simulink model "TopLevelModel"  (R2023a)
settings: Solver=VariableStepAuto  StartTime=0.0  StopTime=inf  RelTol=1e-3
values from neighbouring files (symbols this model uses):
  b = 40.6518    [TopLevelModelParameters.m]
  B1 = 0.0042    [TopLevelModelParameters.m]
  B2 = 0.0084    [TopLevelModelParameters.m]
  J1 = 7e-5    (= 7e-05)    [TopLevelModelParameters.m]
  J2 = 8e-5    (= 8e-05)    [TopLevelModelParameters.m]
  k1 = 2.6552e5    (= 265520)    [TopLevelModelParameters.m]
  k2 = 2.6552e5    (= 265520)    [TopLevelModelParameters.m]
  k3 = 11.777e4    (= 117770)    [TopLevelModelParameters.m]
  Kb = 23e-3    (= 0.023)    [TopLevelModelParameters.m]
  Kt = 23e-3    (= 0.023)    [TopLevelModelParameters.m]
  L = 0.1    [TopLevelModelParameters.m]
  m = 2    [TopLevelModelParameters.m]
  R = 0.71    [TopLevelModelParameters.m]
  r = 0.0194    [TopLevelModelParameters.m]
undefined symbols (not defined in the file or in its folder): J, Kd, Ke
libraries: fl_lib x40, fl_ps_legacy_lib x16, nesl_utility x12, slpidlib x10, SignalEditorBlockLib x4, ee_lib x4, simulink x2
(part 3 of 3)

== system TopLevelModel/Belt2/Subsystem2/Subsystem ==
  Constant : Constant  Value=Kt
  Constant1 : Constant  Value=Ke
  Constant2 : Constant  Value=R
  Divide : Product  Inputs=**/
  Divide1 : Product  Inputs=***/
  Minus3 : Sum  Inputs=+-
  Voltage : DiscretePulseGenerator  PulseType=Time based  Amplitude=12  Period=11  PulseWidth=50  PhaseDelay=2
  Tourque : Outport
  wires:
  Divide1/1 -> Minus3/2
  Divide/1 -> Minus3/1
  Constant/1 -> Divide/2, Divide1/1
  [theta1_dot] -> Divide1/3
  Constant1/1 -> Divide1/2
  Constant2/1 -> Divide1/4, Divide/3
  Minus3/1 -> Tourque/1  "Tourque"
  Voltage/1 -> Divide/1

== system TopLevelModel/Belt3/Subsystem2/DC Motor1 ==
  note: Armature Controlled DC Motor
      |
      | $E_a = R_a \cdot I_a + L_a \cdot \frac{di_a}{dt} + K_b \cdot \frac{d\theta}{dt}$
      | $T_{m} = K_{t} \cdot I_{a}$
  Voltage : Inport
  Velocity : Inport  Port=2
  Constant1 : Constant  Value=R
  Gain1 : Gain  Gain=Kb
  Gain2 : Gain  Gain=1/L
  Gain3 : Gain  Gain=Kt
  Integrator : Integrator
  Product : Product
  Subtract : Sum  Inputs=+--
  Tourque : Outport
  wires:
  Voltage/1 -> Subtract/1
  Integrator/1 -> Product/1, Gain3/1  "i"
  Gain3/1 -> Tourque/1
  Gain1/1 -> Subtract/2
  Velocity/1 -> Gain1/1
  Constant1/1 -> Product/2
  Product/1 -> Subtract/3
  Gain2/1 -> Integrator/1  "i_dot"
  Subtract/1 -> Gain2/1

== system TopLevelModel/Belt3/Subsystem2/Subsystem ==
  Constant : Constant  Value=Kt
  Constant1 : Constant  Value=Ke
  Constant2 : Constant  Value=R
  Divide : Product  Inputs=**/
  Divide1 : Product  Inputs=***/
  Minus3 : Sum  Inputs=+-
  Voltage : DiscretePulseGenerator  PulseType=Time based  Amplitude=12  Period=11  PulseWidth=50  PhaseDelay=2
  Tourque : Outport
  wires:
  Divide1/1 -> Minus3/2
  Divide/1 -> Minus3/1
  Constant/1 -> Divide/2, Divide1/1
  [theta1_dot] -> Divide1/3
  Constant1/1 -> Divide1/2
  Constant2/1 -> Divide1/4, Divide/3
  Minus3/1 -> Tourque/1  "Tourque"
  Voltage/1 -> Divide/1

== system TopLevelModel/Belt4/Subsystem2/DC Motor1 ==
  note: Armature Controlled DC Motor
      |
      | $E_a = R_a \cdot I_a + L_a \cdot \frac{di_a}{dt} + K_b \cdot \frac{d\theta}{dt}$
      | $T_{m} = K_{t} \cdot I_{a}$
  Voltage : Inport
  Velocity : Inport  Port=2
  Constant1 : Constant  Value=R
  Gain1 : Gain  Gain=Kb
  Gain2 : Gain  Gain=1/L
  Gain3 : Gain  Gain=Kt
  Integrator : Integrator
  Product : Product
  Subtract : Sum  Inputs=+--
  Tourque : Outport
  wires:
  Voltage/1 -> Subtract/1
  Integrator/1 -> Product/1, Gain3/1  "i"
  Gain3/1 -> Tourque/1
  Gain1/1 -> Subtract/2
  Velocity/1 -> Gain1/1
  Constant1/1 -> Product/2
  Product/1 -> Subtract/3
  Gain2/1 -> Integrator/1  "i_dot"
  Subtract/1 -> Gain2/1

== system TopLevelModel/Belt4/Subsystem2/Subsystem ==
  Constant : Constant  Value=Kt
  Constant1 : Constant  Value=Ke
  Constant2 : Constant  Value=R
  Divide : Product  Inputs=**/
  Divide1 : Product  Inputs=***/
  Minus3 : Sum  Inputs=+-
  Voltage : DiscretePulseGenerator  PulseType=Time based  Amplitude=12  Period=11  PulseWidth=50  PhaseDelay=2
  Tourque : Outport
  wires:
  Divide1/1 -> Minus3/2
  Divide/1 -> Minus3/1
  Constant/1 -> Divide/2, Divide1/1
  [theta1_dot] -> Divide1/3
  Constant1/1 -> Divide1/2
  Constant2/1 -> Divide1/4, Divide/3
  Minus3/1 -> Tourque/1  "Tourque"
  Voltage/1 -> Divide/1

== system TopLevelModel/Belt5/Subsystem2/DC Motor1 ==
  note: Armature Controlled DC Motor
      |
      | $E_a = R_a \cdot I_a + L_a \cdot \frac{di_a}{dt} + K_b \cdot \frac{d\theta}{dt}$
      | $T_{m} = K_{t} \cdot I_{a}$
  Voltage : Inport
  Velocity : Inport  Port=2
  Constant1 : Constant  Value=R
  Gain1 : Gain  Gain=Kb
  Gain2 : Gain  Gain=1/L
  Gain3 : Gain  Gain=Kt
  Integrator : Integrator
  Product : Product
  Subtract : Sum  Inputs=+--
  Tourque : Outport
  wires:
  Voltage/1 -> Subtract/1
  Integrator/1 -> Product/1, Gain3/1  "i"
  Gain3/1 -> Tourque/1
  Gain1/1 -> Subtract/2
  Velocity/1 -> Gain1/1
  Constant1/1 -> Product/2
  Product/1 -> Subtract/3
  Gain2/1 -> Integrator/1  "i_dot"
  Subtract/1 -> Gain2/1

== system TopLevelModel/Belt5/Subsystem2/Subsystem ==
  Constant : Constant  Value=Kt
  Constant1 : Constant  Value=Ke
  Constant2 : Constant  Value=R
  Divide : Product  Inputs=**/
  Divide1 : Product  Inputs=***/
  Minus3 : Sum  Inputs=+-
  Voltage : DiscretePulseGenerator  PulseType=Time based  Amplitude=12  Period=11  PulseWidth=50  PhaseDelay=2
  Tourque : Outport
  wires:
  Divide1/1 -> Minus3/2
  Divide/1 -> Minus3/1
  Constant/1 -> Divide/2, Divide1/1
  [theta1_dot] -> Divide1/3
  Constant1/1 -> Divide1/2
  Constant2/1 -> Divide1/4, Divide/3
  Minus3/1 -> Tourque/1  "Tourque"
  Voltage/1 -> Divide/1

== system TopLevelModel/Belt6/Subsystem2/DC Motor1 ==
  note: Armature Controlled DC Motor
      |
      | $E_a = R_a \cdot I_a + L_a \cdot \frac{di_a}{dt} + K_b \cdot \frac{d\theta}{dt}$
      | $T_{m} = K_{t} \cdot I_{a}$
  Voltage : Inport
  Velocity : Inport  Port=2
  Constant1 : Constant  Value=R
  Gain1 : Gain  Gain=Kb
  Gain2 : Gain  Gain=1/L
  Gain3 : Gain  Gain=Kt
  Integrator : Integrator
  Product : Product
  Subtract : Sum  Inputs=+--
  Tourque : Outport
  wires:
  Voltage/1 -> Subtract/1
  Integrator/1 -> Product/1, Gain3/1  "i"
  Gain3/1 -> Tourque/1
  Gain1/1 -> Subtract/2
  Velocity/1 -> Gain1/1
  Constant1/1 -> Product/2
  Product/1 -> Subtract/3
  Gain2/1 -> Integrator/1  "i_dot"
  Subtract/1 -> Gain2/1

== system TopLevelModel/Belt6/Subsystem2/Subsystem ==
  Constant : Constant  Value=Kt
  Constant1 : Constant  Value=Ke
  Constant2 : Constant  Value=R
  Divide : Product  Inputs=**/
  Divide1 : Product  Inputs=***/
  Minus3 : Sum  Inputs=+-
  Voltage : DiscretePulseGenerator  PulseType=Time based  Amplitude=12  Period=11  PulseWidth=50  PhaseDelay=2
  Tourque : Outport
  wires:
  Divide1/1 -> Minus3/2
  Divide/1 -> Minus3/1
  Constant/1 -> Divide/2, Divide1/1
  [theta1_dot] -> Divide1/3
  Constant1/1 -> Divide1/2
  Constant2/1 -> Divide1/4, Divide/3
  Minus3/1 -> Tourque/1  "Tourque"
  Voltage/1 -> Divide/1

== system TopLevelModel/Belt7/Subsystem2/DC Motor1 ==
  note: Armature Controlled DC Motor
      |
      | $E_a = R_a \cdot I_a + L_a \cdot \frac{di_a}{dt} + K_b \cdot \frac{d\theta}{dt}$
      | $T_{m} = K_{t} \cdot I_{a}$
  Voltage : Inport
  Velocity : Inport  Port=2
  Constant1 : Constant  Value=R
  Gain1 : Gain  Gain=Kb
  Gain2 : Gain  Gain=1/L
  Gain3 : Gain  Gain=Kt
  Integrator : Integrator
  Product : Product
  Subtract : Sum  Inputs=+--
  Tourque : Outport
  wires:
  Voltage/1 -> Subtract/1
  Integrator/1 -> Product/1, Gain3/1  "i"
  Gain3/1 -> Tourque/1
  Gain1/1 -> Subtract/2
  Velocity/1 -> Gain1/1
  Constant1/1 -> Product/2
  Product/1 -> Subtract/3
  Gain2/1 -> Integrator/1  "i_dot"
  Subtract/1 -> Gain2/1

== system TopLevelModel/Belt7/Subsystem2/Subsystem ==
  Constant : Constant  Value=Kt
  Constant1 : Constant  Value=Ke
  Constant2 : Constant  Value=R
  Divide : Product  Inputs=**/
  Divide1 : Product  Inputs=***/
  Minus3 : Sum  Inputs=+-
  Voltage : DiscretePulseGenerator  PulseType=Time based  Amplitude=12  Period=11  PulseWidth=50  PhaseDelay=2
  Tourque : Outport
  wires:
  Divide1/1 -> Minus3/2
  Divide/1 -> Minus3/1
  Constant/1 -> Divide/2, Divide1/1
  [theta1_dot] -> Divide1/3
  Constant1/1 -> Divide1/2
  Constant2/1 -> Divide1/4, Divide/3
  Minus3/1 -> Tourque/1  "Tourque"
  Voltage/1 -> Divide/1

== system TopLevelModel/Belt8/Subsystem2/DC Motor1 ==
  note: Armature Controlled DC Motor
      |
      | $E_a = R_a \cdot I_a + L_a \cdot \frac{di_a}{dt} + K_b \cdot \frac{d\theta}{dt}$
      | $T_{m} = K_{t} \cdot I_{a}$
  Voltage : Inport
  Velocity : Inport  Port=2
  Constant1 : Constant  Value=R
  Gain1 : Gain  Gain=Kb
  Gain2 : Gain  Gain=1/L
  Gain3 : Gain  Gain=Kt
  Integrator : Integrator
  Product : Product
  Subtract : Sum  Inputs=+--
  Tourque : Outport
  wires:
  Voltage/1 -> Subtract/1
  Integrator/1 -> Product/1, Gain3/1  "i"
  Gain3/1 -> Tourque/1
  Gain1/1 -> Subtract/2
  Velocity/1 -> Gain1/1
  Constant1/1 -> Product/2
  Product/1 -> Subtract/3
  Gain2/1 -> Integrator/1  "i_dot"
  Subtract/1 -> Gain2/1

== system TopLevelModel/Belt8/Subsystem2/Subsystem ==
  Constant : Constant  Value=Kt
  Constant1 : Constant  Value=Ke
  Constant2 : Constant  Value=R
  Divide : Product  Inputs=**/
  Divide1 : Product  Inputs=***/
  Minus3 : Sum  Inputs=+-
  Voltage : DiscretePulseGenerator  PulseType=Time based  Amplitude=12  Period=11  PulseWidth=50  PhaseDelay=2
  Tourque : Outport
  wires:
  Divide1/1 -> Minus3/2
  Divide/1 -> Minus3/1
  Constant/1 -> Divide/2, Divide1/1
  [theta1_dot] -> Divide1/3
  Constant1/1 -> Divide1/2
  Constant2/1 -> Divide1/4, Divide/3
  Minus3/1 -> Tourque/1  "Tourque"
  Voltage/1 -> Divide/1

== system TopLevelModel/Belt9/Subsystem2/DC Motor1 ==
  note: Armature Controlled DC Motor
      |
      | $E_a = R_a \cdot I_a + L_a \cdot \frac{di_a}{dt} + K_b \cdot \frac{d\theta}{dt}$
      | $T_{m} = K_{t} \cdot I_{a}$
  Voltage : Inport
  Velocity : Inport  Port=2
  Constant1 : Constant  Value=R
  Gain1 : Gain  Gain=Kb
  Gain2 : Gain  Gain=1/L
  Gain3 : Gain  Gain=Kt
  Integrator : Integrator
  Product : Product
  Subtract : Sum  Inputs=+--
  Tourque : Outport
  wires:
  Voltage/1 -> Subtract/1
  Integrator/1 -> Product/1, Gain3/1  "i"
  Gain3/1 -> Tourque/1
  Gain1/1 -> Subtract/2
  Velocity/1 -> Gain1/1
  Constant1/1 -> Product/2
  Product/1 -> Subtract/3
  Gain2/1 -> Integrator/1  "i_dot"
  Subtract/1 -> Gain2/1

== system TopLevelModel/Belt9/Subsystem2/Subsystem ==
  Constant : Constant  Value=Kt
  Constant1 : Constant  Value=Ke
  Constant2 : Constant  Value=R
  Divide : Product  Inputs=**/
  Divide1 : Product  Inputs=***/
  Minus3 : Sum  Inputs=+-
  Voltage : DiscretePulseGenerator  PulseType=Time based  Amplitude=12  Period=11  PulseWidth=50  PhaseDelay=2
  Tourque : Outport
  wires:
  Divide1/1 -> Minus3/2
  Divide/1 -> Minus3/1
  Constant/1 -> Divide/2, Divide1/1
  [theta1_dot] -> Divide1/3
  Constant1/1 -> Divide1/2
  Constant2/1 -> Divide1/4, Divide/3
  Minus3/1 -> Tourque/1  "Tourque"
  Voltage/1 -> Divide/1

== system TopLevelModel/Controller/Position/Algorithm and Pulse Generation ==
  note: The reference input defines the required angular position in terms of
      | the number steps. For this stepper, the step size is 1.8 degrees. Hence
      | a demand of 10 steps results in an angle change of 18 degrees.
      | The step rate is set by the Pulse Generator's Pulse rate mask parameter.
  note: Position Controller
  Reference : Inport
  IC Analog Output REV : Subsystem
  IC Analog Output Vref : Subsystem
  Logic2Volts1 : Gain  Gain=5
  Logic2Volts2 : Gain  Gain=5
  Pulse Generator : Subsystem  mask{f=20}
      mask prompts: f "Pulse rate"
  Rate Transition : RateTransition  Deterministic=off
  REV : PMIOPort  Side=Right
  Vref : PMIOPort  Port=2  Side=Right
  wires:
  Logic2Volts1/1 -> IC Analog Output Vref/1(SL)
  Pulse Generator/1(Pulse train) -> Logic2Volts1/1
  Reference/1 -> Rate Transition/1
  Logic2Volts2/1 -> IC Analog Output REV/1(SL)
  Pulse Generator/2(Pulse direction) -> Logic2Volts2/1
  Rate Transition/1 -> Pulse Generator/1(Pulse  demand)
  connections:
  Vref/RConn1 -- IC Analog Output Vref/RConn1
  REV/RConn1 -- IC Analog Output REV/RConn1

== system TopLevelModel/Controller/Speed/Step Rate and Direction ==
  note: The speed controller turns the reference input into an absolute voltage demand for the
      | voltage-controlled pulse generator and sets the reverse flag signal to +5 volts when the
      | speed demand is negative.
  Reference : Inport
  Abs : Abs  SaturateOnIntegerOverflow=off
  Compare To Constant : simulink/Logic and Bit Operations/Compare To Constant  relop=<  const=0  OutDataTypeStr=uint8  ZeroCross=off
  Data Type Conversion : DataTypeConversion  SaturateOnIntegerOverflow=off  RndMeth=Floor
  IC Analog Output REV : Subsystem
  IC Analog Output Vref : Subsystem
  Logic2Volts : Gain  Gain=5
  Max step rate 100/s : Saturate  UpperLimit=100  LowerLimit=0
  StepRate2Volts : Gain  Gain=5/100
  REV : PMIOPort  Side=Right
  Vref : PMIOPort  Port=2  Side=Right
  wires:
  StepRate2Volts/1 -> IC Analog Output Vref/1(SL)
  Max step rate 100/s/1 -> StepRate2Volts/1
  Data Type Conversion/1 -> Logic2Volts/1
  Compare To Constant/1 -> Data Type Conversion/1
  Reference/1 -> Compare To Constant/1, Abs/1
  Abs/1 -> Max step rate 100/s/1
  Logic2Volts/1 -> IC Analog Output REV/1(SL)
  connections:
  REV/RConn1 -- IC Analog Output REV/RConn1
  Vref/RConn1 -- IC Analog Output Vref/RConn1

== system TopLevelModel/Controller/Speed/Voltage-Controlled Pulse Generator ==
  2*pi : fl_ps_legacy_lib/Legacy Physical Signals/Functions/PS Gain  gain=-2*pi
  Controlled Voltage Source : fl_lib/Electrical/Electrical Sources/Controlled Voltage Source
  ERef : fl_lib/Electrical/Electrical Elements/Electrical Reference
  Max step rate =100 : fl_ps_legacy_lib/Legacy Physical Signals/Functions/PS Gain  gain=100
  Normalize to 1 : fl_ps_legacy_lib/Legacy Physical Signals/Functions/PS Gain  gain=1/5
  PS Integrator : fl_ps_legacy_lib/Legacy Physical Signals/Linear Operators/PS Integrator  x0=0
      settings: InternalSimscapePortConfiguration="{\"Bottom\":[],\"Left\":[{\"id\":\"I\",\"label\":\"\",\"type\":\"input\"}],\"Right\":[{\"id\":\"O\",\"label\":\"\",\"type\":\"output\"}],\"Top\":[]}"
  PS Sign : fl_ps_legacy_lib/Legacy Physical Signals/Nonlinear Operators/PS Sign
      settings: InternalSimscapePortConfiguration="{\"Bottom\":[],\"Left\":[{\"id\":\"I\",\"label\":\"\",\"type\":\"input\"}],\"Right\":[{\"id\":\"O\",\"label\":\"\",\"type\":\"output\"}],\"Top\":[]}"
  PS Sine : fl_ps_legacy_lib/Legacy Physical Signals/Functions/PS Math Function  fcn_choice=1
      settings: InternalSimscapePortConfiguration="{\"Bottom\":[],\"Left\":[{\"id\":\"I\",\"label\":\"\",\"type\":\"input\"}],\"Right\":[{\"id\":\"O\",\"label\":\"\",\"type\":\"output\"}],\"Top\":[]}"
  Voltage Sensor : fl_lib/Electrical/Electrical Sensors/Voltage Sensor
  "[0,1]" : fl_ps_legacy_lib/Legacy Physical Signals/Nonlinear Operators/PS Saturation  upper_limit=1  lower_limit=0
      settings: InternalSimscapePortConfiguration="{\"Bottom\":[],\"Left\":[{\"id\":\"I\",\"label\":\"\",\"type\":\"input\"}],\"Right\":[{\"id\":\"O\",\"label\":\"\",\"type\":\"output\"}],\"Top\":[]}"
  logic2volts : fl_ps_legacy_lib/Legacy Physical Signals/Functions/PS Gain  gain=5
  PWM : PMIOPort  Side=Right
  0v : PMIOPort  Port=2  Side=Right
  Vref : PMIOPort  Port=3  Side=Left
  connections:
  PWM/RConn1 -- Controlled Voltage Source/LConn1
  Controlled Voltage Source/RConn2 -- 0v/RConn1
  Vref/RConn1 -- Voltage Sensor/LConn1
  ERef/LConn1 -- Voltage Sensor/RConn2
  Voltage Sensor/RConn1 -- Normalize to 1/LConn1
  Max step rate =100/LConn1 -- Normalize to 1/RConn1
  Max step rate =100/RConn1 -- 2*pi/LConn1
  2*pi/RConn1 -- PS Integrator/LConn1
  PS Integrator/RConn1 -- PS Sine/LConn1
  PS Sign/LConn1 -- PS Sine/RConn1
  "[0,1]"/LConn1 -- PS Sign/RConn1
  "[0,1]"/RConn1 -- logic2volts/LConn1
  logic2volts/RConn1 -- Controlled Voltage Source/RConn1

== system TopLevelModel/Controller1/Position/Algorithm and Pulse Generation ==
  note: The reference input defines the required angular position in terms of
      | the number steps. For this stepper, the step size is 1.8 degrees. Hence
      | a demand of 10 steps results in an angle change of 18 degrees.
      | The step rate is set by the Pulse Generator's Pulse rate mask parameter.
  note: Position Controller
  Reference : Inport
  IC Analog Output REV : Subsystem
  IC Analog Output Vref : Subsystem
  Logic2Volts1 : Gain  Gain=5
  Logic2Volts2 : Gain  Gain=5
  Pulse Generator : Subsystem  mask{f=20}
      mask prompts: f "Pulse rate"
  Rate Transition : RateTransition  Deterministic=off
  REV : PMIOPort  Side=Right
  Vref : PMIOPort  Port=2  Side=Right
  wires:
  Logic2Volts1/1 -> IC Analog Output Vref/1(SL)
  Pulse Generator/1(Pulse train) -> Logic2Volts1/1
  Reference/1 -> Rate Transition/1
  Logic2Volts2/1 -> IC Analog Output REV/1(SL)
  Pulse Generator/2(Pulse direction) -> Logic2Volts2/1
  Rate Transition/1 -> Pulse Generator/1(Pulse  demand)
  connections:
  Vref/RConn1 -- IC Analog Output Vref/RConn1
  REV/RConn1 -- IC Analog Output REV/RConn1

== system TopLevelModel/Controller1/Speed/Step Rate and Direction ==
  note: The speed controller turns the reference input into an absolute voltage demand for the
      | voltage-controlled pulse generator and sets the reverse flag signal to +5 volts when the
      | speed demand is negative.
  Reference : Inport
  Abs : Abs  SaturateOnIntegerOverflow=off
  Compare To Constant : simulink/Logic and Bit Operations/Compare To Constant  relop=<  const=0  OutDataTypeStr=uint8  ZeroCross=off
  Data Type Conversion : DataTypeConversion  SaturateOnIntegerOverflow=off  RndMeth=Floor
  IC Analog Output REV : Subsystem
  IC Analog Output Vref : Subsystem
  Logic2Volts : Gain  Gain=5
  Max step rate 100/s : Saturate  UpperLimit=100  LowerLimit=0
  StepRate2Volts : Gain  Gain=5/100
  REV : PMIOPort  Side=Right
  Vref : PMIOPort  Port=2  Side=Right
  wires:
  StepRate2Volts/1 -> IC Analog Output Vref/1(SL)
  Max step rate 100/s/1 -> StepRate2Volts/1
  Data Type Conversion/1 -> Logic2Volts/1
  Compare To Constant/1 -> Data Type Conversion/1
  Reference/1 -> Compare To Constant/1, Abs/1
  Abs/1 -> Max step rate 100/s/1
  Logic2Volts/1 -> IC Analog Output REV/1(SL)
  connections:
  REV/RConn1 -- IC Analog Output REV/RConn1
  Vref/RConn1 -- IC Analog Output Vref/RConn1

== system TopLevelModel/Controller1/Speed/Voltage-Controlled Pulse Generator ==
  2*pi : fl_ps_legacy_lib/Legacy Physical Signals/Functions/PS Gain  gain=-2*pi
  Controlled Voltage Source : fl_lib/Electrical/Electrical Sources/Controlled Voltage Source
  ERef : fl_lib/Electrical/Electrical Elements/Electrical Reference
  Max step rate =100 : fl_ps_legacy_lib/Legacy Physical Signals/Functions/PS Gain  gain=100
  Normalize to 1 : fl_ps_legacy_lib/Legacy Physical Signals/Functions/PS Gain  gain=1/5
  PS Integrator : fl_ps_legacy_lib/Legacy Physical Signals/Linear Operators/PS Integrator  x0=0
      settings: InternalSimscapePortConfiguration="{\"Bottom\":[],\"Left\":[{\"id\":\"I\",\"label\":\"\",\"type\":\"input\"}],\"Right\":[{\"id\":\"O\",\"label\":\"\",\"type\":\"output\"}],\"Top\":[]}"
  PS Sign : fl_ps_legacy_lib/Legacy Physical Signals/Nonlinear Operators/PS Sign
      settings: InternalSimscapePortConfiguration="{\"Bottom\":[],\"Left\":[{\"id\":\"I\",\"label\":\"\",\"type\":\"input\"}],\"Right\":[{\"id\":\"O\",\"label\":\"\",\"type\":\"output\"}],\"Top\":[]}"
  PS Sine : fl_ps_legacy_lib/Legacy Physical Signals/Functions/PS Math Function  fcn_choice=1
      settings: InternalSimscapePortConfiguration="{\"Bottom\":[],\"Left\":[{\"id\":\"I\",\"label\":\"\",\"type\":\"input\"}],\"Right\":[{\"id\":\"O\",\"label\":\"\",\"type\":\"output\"}],\"Top\":[]}"
  Voltage Sensor : fl_lib/Electrical/Electrical Sensors/Voltage Sensor
  "[0,1]" : fl_ps_legacy_lib/Legacy Physical Signals/Nonlinear Operators/PS Saturation  upper_limit=1  lower_limit=0
      settings: InternalSimscapePortConfiguration="{\"Bottom\":[],\"Left\":[{\"id\":\"I\",\"label\":\"\",\"type\":\"input\"}],\"Right\":[{\"id\":\"O\",\"label\":\"\",\"type\":\"output\"}],\"Top\":[]}"
  logic2volts : fl_ps_legacy_lib/Legacy Physical Signals/Functions/PS Gain  gain=5
  PWM : PMIOPort  Side=Right
  0v : PMIOPort  Port=2  Side=Right
  Vref : PMIOPort  Port=3  Side=Left
  connections:
  PWM/RConn1 -- Controlled Voltage Source/LConn1
  Controlled Voltage Source/RConn2 -- 0v/RConn1
  Vref/RConn1 -- Voltage Sensor/LConn1
  ERef/LConn1 -- Voltage Sensor/RConn2
  Voltage Sensor/RConn1 -- Normalize to 1/LConn1
  Max step rate =100/LConn1 -- Normalize to 1/RConn1
  Max step rate =100/RConn1 -- 2*pi/LConn1
  2*pi/RConn1 -- PS Integrator/LConn1
  PS Integrator/RConn1 -- PS Sine/LConn1
  PS Sign/LConn1 -- PS Sine/RConn1
  "[0,1]"/LConn1 -- PS Sign/RConn1
  "[0,1]"/RConn1 -- logic2volts/LConn1
  logic2volts/RConn1 -- Controlled Voltage Source/RConn1

== system TopLevelModel/Controller/Position/Algorithm and Pulse Generation/IC Analog Output REV ==
  SL : Inport
  Controlled Voltage Source : fl_lib/Electrical/Electrical Sources/Controlled Voltage Source
  ERef : fl_lib/Electrical/Electrical Elements/Electrical Reference
  Simulink-PS Converter : nesl_utility/Simulink-PS Converter  PhysicalDomain=network_engine_domain  SubClassName=ps_input  LeftPortType=input  RightPortType=output  PseudoPeriodic=off  Frequencies=[]  NoiseDistribution=none  NoiseParameters=[]  Unit=V  AffineConversion=off  FilteringAndDerivatives=zero  SimscapeFilterOrder=1  InputFilterTimeConstant=.001  UdotUserProvided=0
  V : PMIOPort  Side=Right
  wires:
  SL/1 -> Simulink-PS Converter/1
  connections:
  ERef/LConn1 -- Controlled Voltage Source/RConn2
  V/RConn1 -- Controlled Voltage Source/LConn1
  Simulink-PS Converter/RConn1 -- Controlled Voltage Source/RConn1

== system TopLevelModel/Controller/Position/Algorithm and Pulse Generation/IC Analog Output Vref ==
  SL : Inport
  Controlled Voltage Source : fl_lib/Electrical/Electrical Sources/Controlled Voltage Source
  ERef : fl_lib/Electrical/Electrical Elements/Electrical Reference
  Simulink-PS Converter : nesl_utility/Simulink-PS Converter  PhysicalDomain=network_engine_domain  SubClassName=ps_input  LeftPortType=input  RightPortType=output  PseudoPeriodic=off  Frequencies=[]  NoiseDistribution=none  NoiseParameters=[]  Unit=V  AffineConversion=off  FilteringAndDerivatives=zero  SimscapeFilterOrder=1  InputFilterTimeConstant=.001  UdotUserProvided=0
  V : PMIOPort  Side=Right
  wires:
  SL/1 -> Simulink-PS Converter/1
  connections:
  Simulink-PS Converter/RConn1 -- Controlled Voltage Source/RConn1
  V/RConn1 -- Controlled Voltage Source/LConn1
  ERef/LConn1 -- Controlled Voltage Source/RConn2

== system TopLevelModel/Controller/Position/Algorithm and Pulse Generation/Pulse Generator ==
  Pulse  demand : Inport  SampleTime=1/f
  -1 : Gain  Gain=-1
  Abs : Abs  SaturateOnIntegerOverflow=off
  Product : Product  InputSameDT=on  SaturateOnIntegerOverflow=on  OutDataTypeStr=Inherit: Same as first input
  Pulse Generator : Subsystem
  Rate Transition : RateTransition  Deterministic=off
  Saturation : Saturate  UpperLimit=1  LowerLimit=-1
  Sign : Signum
  Sum : Sum  Inputs=|+-
  Sum1 : Sum  Inputs=|++
  "Unit Delay, sample time 1/f" : UnitDelay  SampleTime=1/f  HasFrameUpgradeWarning=on
  "[0,1]" : Saturate  UpperLimit=1  LowerLimit=0
  Pulse train : Outport  VectorParamsAs1DForOutWhenUnconnected=off
  Pulse direction : Outport  Port=2  VectorParamsAs1DForOutWhenUnconnected=off
  wires:
  "[0,1]"/1 -> Pulse direction/1
  -1/1 -> Sign/1
  "Unit Delay, sample time 1/f"/1 -> Sum/2, Sum1/2
  Pulse  demand/1 -> Sum/1
  Sum/1 -> -1/1, Saturation/1
  Saturation/1 -> Sum1/1, Abs/1
  Sum1/1 -> "Unit Delay, sample time 1/f"/1
  Sign/1 -> "[0,1]"/1
  Product/1 -> Pulse train/1
  Abs/1 -> Rate Transition/1
  Pulse Generator/1(p) -> Product/2
  Rate Transition/1 -> Product/1

== system TopLevelModel/Controller/Speed/Step Rate and Direction/IC Analog Output REV ==
  SL : Inport
  Controlled Voltage Source : fl_lib/Electrical/Electrical Sources/Controlled Voltage Source
  ERef : fl_lib/Electrical/Electrical Elements/Electrical Reference
  Simulink-PS Converter : nesl_utility/Simulink-PS Converter  PhysicalDomain=network_engine_domain  SubClassName=ps_input  LeftPortType=input  RightPortType=output  PseudoPeriodic=off  Frequencies=[]  NoiseDistribution=none  NoiseParameters=[]  Unit=V  AffineConversion=off  FilteringAndDerivatives=zero  SimscapeFilterOrder=1  InputFilterTimeConstant=.001  UdotUserProvided=0
  V : PMIOPort  Side=Right
  wires:
  SL/1 -> Simulink-PS Converter/1
  connections:
  Simulink-PS Converter/RConn1 -- Controlled Voltage Source/RConn1
  V/RConn1 -- Controlled Voltage Source/LConn1
  ERef/LConn1 -- Controlled Voltage Source/RConn2

== system TopLevelModel/Controller/Speed/Step Rate and Direction/IC Analog Output Vref ==
  SL : Inport
  Controlled Voltage Source : fl_lib/Electrical/Electrical Sources/Controlled Voltage Source
  ERef : fl_lib/Electrical/Electrical Elements/Electrical Reference
  Simulink-PS Converter : nesl_utility/Simulink-PS Converter  PhysicalDomain=network_engine_domain  SubClassName=ps_input  LeftPortType=input  RightPortType=output  PseudoPeriodic=off  Frequencies=[]  NoiseDistribution=none  NoiseParameters=[]  Unit=V  AffineConversion=off  FilteringAndDerivatives=zero  SimscapeFilterOrder=1  InputFilterTimeConstant=.001  UdotUserProvided=0
  V : PMIOPort  Side=Right
  wires:
  SL/1 -> Simulink-PS Converter/1
  connections:
  ERef/LConn1 -- Controlled Voltage Source/RConn2
  V/RConn1 -- Controlled Voltage Source/LConn1
  Simulink-PS Converter/RConn1 -- Controlled Voltage Source/RConn1

== system TopLevelModel/Controller1/Position/Algorithm and Pulse Generation/IC Analog Output REV ==
  SL : Inport
  Controlled Voltage Source : fl_lib/Electrical/Electrical Sources/Controlled Voltage Source
  ERef : fl_lib/Electrical/Electrical Elements/Electrical Reference
  Simulink-PS Converter : nesl_utility/Simulink-PS Converter  PhysicalDomain=network_engine_domain  SubClassName=ps_input  LeftPortType=input  RightPortType=output  PseudoPeriodic=off  Frequencies=[]  NoiseDistribution=none  NoiseParameters=[]  Unit=V  AffineConversion=off  FilteringAndDerivatives=zero  SimscapeFilterOrder=1  InputFilterTimeConstant=.001  UdotUserProvided=0
  V : PMIOPort  Side=Right
  wires:
  SL/1 -> Simulink-PS Converter/1
  connections:
  ERef/LConn1 -- Controlled Voltage Source/RConn2
  V/RConn1 -- Controlled Voltage Source/LConn1
  Simulink-PS Converter/RConn1 -- Controlled Voltage Source/RConn1

== system TopLevelModel/Controller1/Position/Algorithm and Pulse Generation/IC Analog Output Vref ==
  SL : Inport
  Controlled Voltage Source : fl_lib/Electrical/Electrical Sources/Controlled Voltage Source
  ERef : fl_lib/Electrical/Electrical Elements/Electrical Reference
  Simulink-PS Converter : nesl_utility/Simulink-PS Converter  PhysicalDomain=network_engine_domain  SubClassName=ps_input  LeftPortType=input  RightPortType=output  PseudoPeriodic=off  Frequencies=[]  NoiseDistribution=none  NoiseParameters=[]  Unit=V  AffineConversion=off  FilteringAndDerivatives=zero  SimscapeFilterOrder=1  InputFilterTimeConstant=.001  UdotUserProvided=0
  V : PMIOPort  Side=Right
  wires:
  SL/1 -> Simulink-PS Converter/1
  connections:
  Simulink-PS Converter/RConn1 -- Controlled Voltage Source/RConn1
  V/RConn1 -- Controlled Voltage Source/LConn1
  ERef/LConn1 -- Controlled Voltage Source/RConn2

== system TopLevelModel/Controller1/Position/Algorithm and Pulse Generation/Pulse Generator ==
  Pulse  demand : Inport  SampleTime=1/f
  -1 : Gain  Gain=-1
  Abs : Abs  SaturateOnIntegerOverflow=off
  Product : Product  InputSameDT=on  SaturateOnIntegerOverflow=on  OutDataTypeStr=Inherit: Same as first input
  Pulse Generator : Subsystem
  Rate Transition : RateTransition  Deterministic=off
  Saturation : Saturate  UpperLimit=1  LowerLimit=-1
  Sign : Signum
  Sum : Sum  Inputs=|+-
  Sum1 : Sum  Inputs=|++
  "Unit Delay, sample time 1/f" : UnitDelay  SampleTime=1/f  HasFrameUpgradeWarning=on
  "[0,1]" : Saturate  UpperLimit=1  LowerLimit=0
  Pulse train : Outport  VectorParamsAs1DForOutWhenUnconnected=off
  Pulse direction : Outport  Port=2  VectorParamsAs1DForOutWhenUnconnected=off
  wires:
  "[0,1]"/1 -> Pulse direction/1
  -1/1 -> Sign/1
  "Unit Delay, sample time 1/f"/1 -> Sum/2, Sum1/2
  Pulse  demand/1 -> Sum/1
  Sum/1 -> -1/1, Saturation/1
  Saturation/1 -> Sum1/1, Abs/1
  Sum1/1 -> "Unit Delay, sample time 1/f"/1
  Sign/1 -> "[0,1]"/1
  Product/1 -> Pulse train/1
  Abs/1 -> Rate Transition/1
  Pulse Generator/1(p) -> Product/2
  Rate Transition/1 -> Product/1

== system TopLevelModel/Controller1/Speed/Step Rate and Direction/IC Analog Output REV ==
  SL : Inport
  Controlled Voltage Source : fl_lib/Electrical/Electrical Sources/Controlled Voltage Source
  ERef : fl_lib/Electrical/Electrical Elements/Electrical Reference
  Simulink-PS Converter : nesl_utility/Simulink-PS Converter  PhysicalDomain=network_engine_domain  SubClassName=ps_input  LeftPortType=input  RightPortType=output  PseudoPeriodic=off  Frequencies=[]  NoiseDistribution=none  NoiseParameters=[]  Unit=V  AffineConversion=off  FilteringAndDerivatives=zero  SimscapeFilterOrder=1  InputFilterTimeConstant=.001  UdotUserProvided=0
  V : PMIOPort  Side=Right
  wires:
  SL/1 -> Simulink-PS Converter/1
  connections:
  Simulink-PS Converter/RConn1 -- Controlled Voltage Source/RConn1
  V/RConn1 -- Controlled Voltage Source/LConn1
  ERef/LConn1 -- Controlled Voltage Source/RConn2

== system TopLevelModel/Controller1/Speed/Step Rate and Direction/IC Analog Output Vref ==
  SL : Inport
  Controlled Voltage Source : fl_lib/Electrical/Electrical Sources/Controlled Voltage Source
  ERef : fl_lib/Electrical/Electrical Elements/Electrical Reference
  Simulink-PS Converter : nesl_utility/Simulink-PS Converter  PhysicalDomain=network_engine_domain  SubClassName=ps_input  LeftPortType=input  RightPortType=output  PseudoPeriodic=off  Frequencies=[]  NoiseDistribution=none  NoiseParameters=[]  Unit=V  AffineConversion=off  FilteringAndDerivatives=zero  SimscapeFilterOrder=1  InputFilterTimeConstant=.001  UdotUserProvided=0
  V : PMIOPort  Side=Right
  wires:
  SL/1 -> Simulink-PS Converter/1
  connections:
  ERef/LConn1 -- Controlled Voltage Source/RConn2
  V/RConn1 -- Controlled Voltage Source/LConn1
  Simulink-PS Converter/RConn1 -- Controlled Voltage Source/RConn1

== system TopLevelModel/Controller/Position/Algorithm and Pulse Generation/Pulse Generator/Pulse Generator ==
  -1 : Gain  Gain=0.5
  Constant : Constant  SampleTime=1/(2*f)
  Gain : Gain  Gain=-1
  Sum : Sum  Inputs=|++
  "Unit Delay, sample time 1/2*f)" : UnitDelay  InitialCondition=-1  SampleTime=1/(2*f)  HasFrameUpgradeWarning=on
  p : Outport  VectorParamsAs1DForOutWhenUnconnected=off
  wires:
  "Unit Delay, sample time 1/2*f)"/1 -> Gain/1, Sum/1
  Gain/1 -> "Unit Delay, sample time 1/2*f)"/1
  Constant/1 -> Sum/2
  Sum/1 -> -1/1
  -1/1 -> p/1

== system TopLevelModel/Controller1/Position/Algorithm and Pulse Generation/Pulse Generator/Pulse Generator ==
  -1 : Gain  Gain=0.5
  Constant : Constant  SampleTime=1/(2*f)
  Gain : Gain  Gain=-1
  Sum : Sum  Inputs=|++
  "Unit Delay, sample time 1/2*f)" : UnitDelay  InitialCondition=-1  SampleTime=1/(2*f)  HasFrameUpgradeWarning=on
  p : Outport  VectorParamsAs1DForOutWhenUnconnected=off
  wires:
  "Unit Delay, sample time 1/2*f)"/1 -> Gain/1, Sum/1
  Gain/1 -> "Unit Delay, sample time 1/2*f)"/1
  Constant/1 -> Sum/2
  Sum/1 -> -1/1
  -1/1 -> p/1

== stateflow chart TopLevelModel/Sensors Logic ==
  state Motor9
    entry:
    V9=1;
  state Motor8
    entry:
    V8=1;
  state Motor7
    entry:
    V7=1;
  state Motor1
    entry:
    V1=1;
  state Motor2
    entry:
    V2=1;
  state Motor6
    entry:
    V6=1;
  state Stationery
    entry:
    V1=0; V2=0; V3=0; V4=0; V5=0; V6=0;
    V7=0; V8=0; V9=0;
  state Motor3
    entry:
    V3=1;
  state Motor5
    entry:
    V5=1;
  state Motor4
    entry:
    V4=1;
  Stationery -> Motor8 [order 8] : [XTheta==144&&YTheta==144]
  Motor8 -> Stationery : [Belt8==1]
  Stationery -> Motor9 [order 9] : [XTheta==162&&YTheta==162]
  Motor9 -> Stationery : [Belt9==1]
  Motor7 -> Stationery : [Belt7==1]
  Stationery -> Motor7 [order 7] : [XTheta==126&&YTheta==126]
  Stationery -> Motor1 [order 1] : [XTheta>17&&YTheta>17&&counter<1]{counter=counter+1}
  Motor1 -> Stationery : [Belt1==1]
  Stationery -> Motor2 [order 2] : [XTheta==36&&YTheta==36]
  Motor6 -> Stationery : [Belt6==1]
  Motor2 -> Stationery : [Belt2==1]
  Stationery -> Motor6 [order 6] : [XTheta==108&&YTheta==108]
  Motor5 -> Stationery : [Belt5==1]
  Stationery -> Motor5 [order 5] : [XTheta==90&&YTheta==90]
  (default) -> Stationery : {counter=0;}
  Motor4 -> Stationery : [Belt4==1]
  Stationery -> Motor4 [order 4] : [XTheta==72&&YTheta==72]
  Motor3 -> Stationery : [Belt3==1]
  Stationery -> Motor3 [order 3] : [XTheta==54&&YTheta==54]
  data: Belt1 input; Belt2 input; Belt3 input; Belt4 input; Belt5 input; Belt6 input; Belt7 input; Belt8 input; Belt9 input; XTheta input; YTheta input; V1 output; V2 output; V3 output; V4 output; V5 output; V6 output; V7 output; V8 output; V9 output; counter output double

== matlab function TopLevelModel/MATLAB Function ==
  data: x output; meal input; y output
function [x, y] = mealSelector(meal)
    % Initialize variables
    x = 0;
    y = 0;

    % Check the chosen meal
    switch meal
        case 1
            x = 10;
            y = 10;
        case 2
            x = 20;
            y = 20;
        case 3
            x = 30;
            y = 30;
        case 4
            x = 40;
            y = 40;
        case 5
            x = 50;
            y = 50;
        case 6
            x = 60;
            y = 60;
        case 7
            x = 70;
            y = 70;
        case 8
            x = 80;
            y = 80;
        case 9
            x = 90;
            y = 90;
        otherwise
            disp('Invalid option. No change to x and y.');
    end
end

== stateflow chart TopLevelModel/Sensors ==
  state Stationery
    entry:
    Voltage=0;
  state Motion
    entry:
    Voltage=1;
  (default) -> Stationery
  Stationery -> Motion : [Crane==1]
  Motion -> Stationery : [Belt==1]
  data: Crane input; Belt input; Voltage output

== stateflow chart TopLevelModel/SteppermotorsLogic ==
  state FetchingM1
    during:
    x==1; y==1;
  state FetchingM2
    during:
    x==2; y==2;
  state ToTheGate
    during:
    x==30;y==30
    state Homing
      during:
      x==0; y==0;
    ToTheGate -> Homing : [payloadClear==1]{x==0&y==0}
    (default) -> Homing
  state FetchingM9
    during:
    x==9; y==9;
  state FetchingM3
    during:
    x==3; y==3;
  state FetchingM8
    during:
    x==8; y==8;
  state FetchingM4
    during:
    x==4; y==4;
  state FetchingM7
    during:
    x==7; y==7;
  state FetchingM5
    during:
    x==5; y==5;
  state FetchingM6
    during:
    x==6; y==6;
  FetchingM1 -> ToTheGate : [payloadOn==1]{x==30&y==30}
  Homing -> FetchingM1 [order 1] : [x==1&y==1]
  FetchingM2 -> ToTheGate : [payloadOn==1]{x==30&y==30}
  Homing -> FetchingM2 [order 2] : [x==2&y==2]
  FetchingM9 -> ToTheGate : [payloadOn==1]{x==30&y==30}
  Homing -> FetchingM9 [order 9] : [x==9&y==9]
  FetchingM3 -> ToTheGate : [payloadOn==1]{x==30&y==30}
  Homing -> FetchingM3 [order 3] : [x==3&y==3]
  FetchingM8 -> ToTheGate : [payloadOn==1]{x==30&y==30}
  Homing -> FetchingM8 [order 8] : [x==8&y==8]
  FetchingM4 -> ToTheGate : [payloadOn==1]{x==30&y==30}
  Homing -> FetchingM4 [order 4] : [x==4&y==4]
  Homing -> FetchingM7 [order 7] : [x==7&y==7]
  Homing -> FetchingM6 [order 6] : [x==6&y==6]
  Homing -> FetchingM5 [order 5] : [x==5&y==5]
  FetchingM7 -> ToTheGate : [payloadOn==1]{x==30&y==30}
  FetchingM5 -> ToTheGate : [payloadOn==1]{x==30&y==30}
  FetchingM6 -> ToTheGate : [payloadOn==1]{x==30&y==30}
  data: payloadClear input; payloadOn input; x input; y input
